simulink model "rule_DJ"  (R2021a)
settings: Solver=FixedStepAuto  StartTime=0.0  StopTime=8.9  FixedStep=1/30  RelTol=1e-3
values from neighbouring files (symbols this model uses):
  y = zeros(10,4)    [simulate.m]
libraries: simulink x17
(part 1 of 3)
settings Model: NumberOfSteps=5  Creator=80720  LastModifiedBy=Administrator
settings SolverCC: AlgebraicLoopSolver=TrustRegion
settings DataIOCC: ReturnWorkspaceOutputs=off
settings DebuggingCC: SFMachineParentedDataDiag=warning  ArithmeticOperatorsInVariantConditions=warning
settings SFSimCC: SimUseLocalCustomCode=off  CustomCodeUndefinedFunction=UseInterfaceOnly
settings RTWCC: RTWUseLocalCustomCode=off

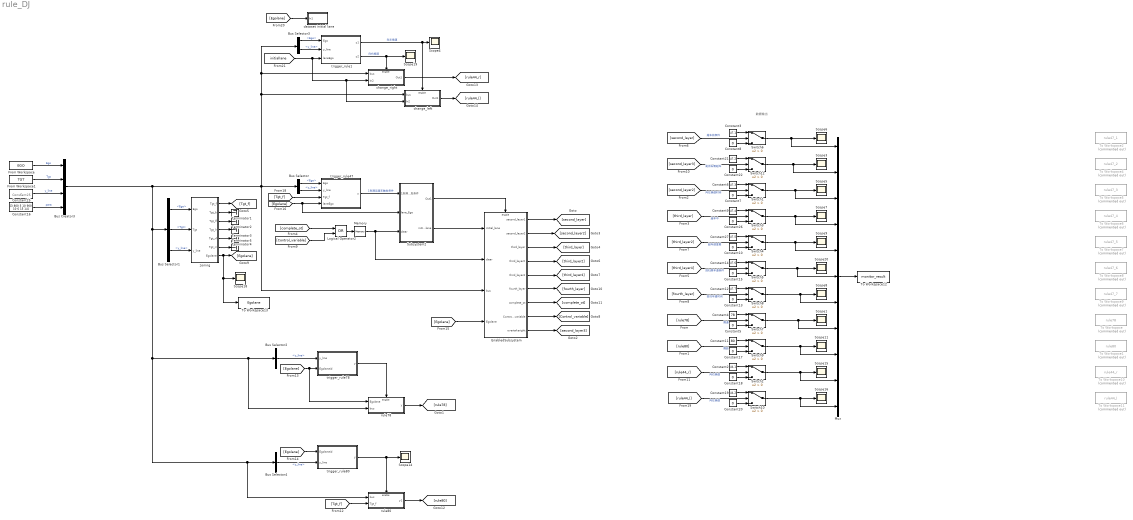
== system rule_DJ ==
  note: Constant25
  note: 数据输出
  Bus Creator3 : BusCreator  Inputs=4
  Bus Selector : BusSelector  OutputSignals=Ego,y_line
  Bus Selector1 : BusSelector  OutputSignals=Ego,Tgt,y_line
  Bus Selector2 : BusSelector  OutputSignals=y_line
  Bus Selector3 : BusSelector  OutputSignals=Ego,y_line
  Bus Selector4 : BusSelector  OutputSignals=y_line
  Constant{5,7..8,10,13,15,17..18,20,22,26} (11 alike) : Constant  Value=0
  Constant11 : Constant  Value=80
  Constant12 : Constant  Value=47.7
  Constant14 : Constant  Value=47.6
  Constant16 : Constant  Value=[3 800 5 10 900 10 6 15 14]
  Constant19 : Constant  Value=44.2
  Constant2 : Constant  Value=44.1
  Constant21 : Constant  Value=47.2
  Constant25 : Constant  Value=y
  Constant27 : Constant  Value=47.5
  Constant3 : Constant  Value=47.1
  Constant4 : Constant  Value=78
  Constant6 : Constant  Value=47.3
  Constant9 : Constant  Value=47.4
  EnabledSubsystem : Subsystem  TreatAsAtomicUnit=on
  From Workspace : FromWorkspace  VariableName=EGO  OutDataTypeStr=Bus: EgoBUS
  From Workspace1 : FromWorkspace  VariableName=TGT  OutDataTypeStr=Bus: TgtBUS
  Logical Operator2 : Logic  Operator=OR  AllPortsSameDT=off  OutDataTypeStr=boolean
  Memory : Memory
  Mux : Mux  Inputs=11
  Scope{1,3..9,11,14..16,18..20} (15 alike) : Scope
  Subsystem2 : Subsystem
  Switch{1..10,12} (11 alike) : Switch  Criteria=u2 > Threshold
  Terminator{1..5} (5 alike) : Terminator
  To Workspace : ToWorkspace  Commented=on  VariableName=rule78  SaveFormat=Timeseries  SampleTime=-1
  To Workspace1 : ToWorkspace  Commented=on  VariableName=rule80  SaveFormat=Timeseries  SampleTime=-1
  To Workspace10 : ToWorkspace  Commented=on  VariableName=rule44_r  SaveFormat=Timeseries  SampleTime=-1
  To Workspace11 : ToWorkspace  Commented=on  VariableName=rule44_l  SaveFormat=Timeseries  SampleTime=-1
  To Workspace12 : ToWorkspace  VariableName=monitor_result  SaveFormat=Timeseries  SampleTime=-1
  To Workspace13 : ToWorkspace  VariableName=Egolane  SaveFormat=Timeseries  SampleTime=-1
  To Workspace2 : ToWorkspace  Commented=on  VariableName=rule47_1  SaveFormat=Timeseries  SampleTime=-1
  To Workspace4 : ToWorkspace  Commented=on  VariableName=rule47_2  SaveFormat=Timeseries  SampleTime=-1
  To Workspace5 : ToWorkspace  Commented=on  VariableName=rule47_3  SaveFormat=Timeseries  SampleTime=-1
  To Workspace6 : ToWorkspace  Commented=on  VariableName=rule47_4  SaveFormat=Timeseries  SampleTime=-1
  To Workspace7 : ToWorkspace  Commented=on  VariableName=rule47_5  SaveFormat=Timeseries  SampleTime=-1
  To Workspace8 : ToWorkspace  Commented=on  VariableName=rule47_6  SaveFormat=Timeseries  SampleTime=-1
  To Workspace9 : ToWorkspace  Commented=on  VariableName=rule47_7  SaveFormat=Timeseries  SampleTime=-1
  change_left : Subsystem  TreatAsAtomicUnit=on
  change_right : Subsystem  TreatAsAtomicUnit=on
  dataset initial lane : Subsystem
  rule78 : Subsystem  TreatAsAtomicUnit=on
  rule80 : Subsystem  TreatAsAtomicUnit=on
  trigger_rule1 : MATLAB Function  TreatAsAtomicUnit=on
  trigger_rule47 : MATLAB Function  TreatAsAtomicUnit=on
  trigger_rule78 : MATLAB Function  TreatAsAtomicUnit=on
  trigger_rule80 : MATLAB Function  TreatAsAtomicUnit=on
  zoning : MATLAB Function  TreatAsAtomicUnit=on
  wires:
  Bus Selector/2 -> trigger_rule47/2(y_line)  "<y_line>"
  Bus Selector/1 -> trigger_rule47/1(Ego)  "<Ego>"
  trigger_rule47/1(y) -> Subsystem2/1(1则满足超车触发条件)  "1则满足超车触发条件"
  Subsystem2/1(Out1) -> EnabledSubsystem/Enable
  Subsystem2/2(initial_lane) -> EnabledSubsystem/1(initial_lane)
  EnabledSubsystem/1(second_layer1) -> [second_layer]
  EnabledSubsystem/3(third_layer) -> [third_layer]
  EnabledSubsystem/4(third_layer2) -> [third_layer2]
  EnabledSubsystem/5(third_layer4) -> [third_layer4]
  EnabledSubsystem/6(fourth_layer) -> [fourth_layer]
  EnabledSubsystem/7(complete_ot) -> [complete_ot]
  EnabledSubsystem/8(Control_variable) -> [Control_variable]
  Constant22/1 -> Switch12/3
  Constant3/1 -> Switch6/1
  Constant13/1 -> Switch8/3
  [fourth_layer] -> Switch8/2  "回归车道时间"
  Constant15/1 -> Switch5/3
  Constant9/1 -> Switch3/1
  Constant21/1 -> Switch12/1
  Switch12/1 -> Mux/2, Scope3/1
  [second_layer3] -> Switch12/2  "是否右侧超车"
  [third_layer2] -> Switch4/2  "超车速度差"
  Constant27/1 -> Switch4/1
  Constant12/1 -> Switch8/1
  Constant10/1 -> Switch4/3
  [third_layer] -> Switch3/2  "超车中"
  [second_layer2] -> Switch1/2  "向左换道时间"
  Constant26/1 -> Switch3/3
  Constant6/1 -> Switch1/1
  Constant7/1 -> Switch1/3
  [second_layer] -> Switch6/2  "超车前条件"
  Constant14/1 -> Switch5/1
  [third_layer4] -> Switch5/2  "回归原车道条件"
  Constant8/1 -> Switch6/3
  Switch6/1 -> Mux/1, Scope6/1
  EnabledSubsystem/9(overtakeright) -> [second_layer3]
  EnabledSubsystem/2(second_layer2) -> [second_layer2]
  From Workspace1/1 -> Bus Creator3/2  "Tgt"
  Constant25/1 -> Bus Creator3/3  "y_line"
  Constant16/1 -> Bus Creator3/4  "para"
  rule78/1(y) -> [rule78]
  trigger_rule78/1(y) -> rule78/Enable
  Bus Selector2/1 -> trigger_rule78/1(y_line)  "<y_line>"
  Bus Selector1/1 -> zoning/1(Ego)  "<Ego>"
  Bus Selector1/2 -> zoning/2(Tgt)  "<Tgt>"
  Bus Selector1/3 -> zoning/3(y_line)  "<y_line>"
  zoning/1(Tgt_f) -> [Tgt_f]
  zoning/2(Tgt_b) -> Terminator1/1
  zoning/3(Tgt_lf) -> Terminator2/1
  zoning/4(Tgt_lr) -> Terminator3/1
  zoning/5(Tgt_rf) -> Terminator4/1
  zoning/6(Tgt_rr) -> Terminator5/1
  [Tgt_f] -> trigger_rule47/3(Tgt_f)
  [Control_variable] -> Logical Operator2/2
  [complete_ot] -> Logical Operator2/1
  Logical Operator2/1 -> Memory/1
  Memory/1 -> EnabledSubsystem/2(clear), Subsystem2/3(clear)
  Bus Selector4/1 -> trigger_rule80/2(y_line)  "<y_line>"
  trigger_rule80/1(y) -> rule80/Enable, Scope14/1
  [Tgt_f] -> rule80/2(Tgt_f)
  zoning/7(Egolane) -> To Workspace13/1, Scope18/1, [Egolane]
  [Egolane] -> rule78/1(Egolane), trigger_rule78/2(Egolaneid)
  [Egolane] -> trigger_rule80/1(Egolaneid)
  [Egolane] -> Subsystem2/2(lane_Ego), trigger_rule47/4(laneEgo)
  [Egolane] -> EnabledSubsystem/4(Egolane)
  From Workspace/1 -> Bus Creator3/1  "Ego"
  Bus Creator3/1 -> Bus Selector1/1, rule80/1(bus), Bus Selector4/1, rule78/2(bus), Bus Selector2/1, change_right/1(bus), Bus Selector3/1, change_left/1(bus), Bus Selector/1, EnabledSubsystem/3(bus)
  Bus Selector3/1 -> trigger_rule1/1(Ego)  "<Ego>"
  Bus Selector3/2 -> trigger_rule1/2(y_line)  "<y_line>"
  [initiallane] -> change_left/2(In2), change_right/2(In2), trigger_rule1/3(laneEgo)
  trigger_rule1/1(y1) -> change_left/Enable, Scope4/1  "向左换道"
  trigger_rule1/2(y2) -> change_right/Enable, Scope19/1  "向右换道"
  Switch3/1 -> Mux/4, Scope7/1
  Switch4/1 -> Mux/5, Scope9/1
  Switch5/1 -> Mux/6, Scope20/1
  Switch8/1 -> Mux/7, Scope8/1
  Switch1/1 -> Mux/3, Scope5/1
  Constant5/1 -> Switch7/3
  Constant4/1 -> Switch7/1
  [rule78] -> Switch7/2  "限速"
  rule80/1(y1) -> [rule80]
  Constant11/1 -> Switch9/1
  [rule80] -> Switch9/2  "限距"
  Constant17/1 -> Switch9/3
  Switch7/1 -> Mux/8, Scope1/1
  Switch9/1 -> Mux/9, Scope11/1
  change_right/1(Out1) -> [rule44_r]
  change_left/1(Out1) -> [rule44_l]
  Switch2/1 -> Mux/10, Scope15/1
  Constant2/1 -> Switch2/1
  Constant18/1 -> Switch2/3
  [rule44_r] -> Switch2/2  "向右换道"
  Switch10/1 -> Mux/11, Scope16/1
  Constant19/1 -> Switch10/1
  Constant20/1 -> Switch10/3
  [rule44_l] -> Switch10/2  "向左换道"
  Mux/1 -> To Workspace12/1
  [Egolane] -> dataset initial lane/1(In1)

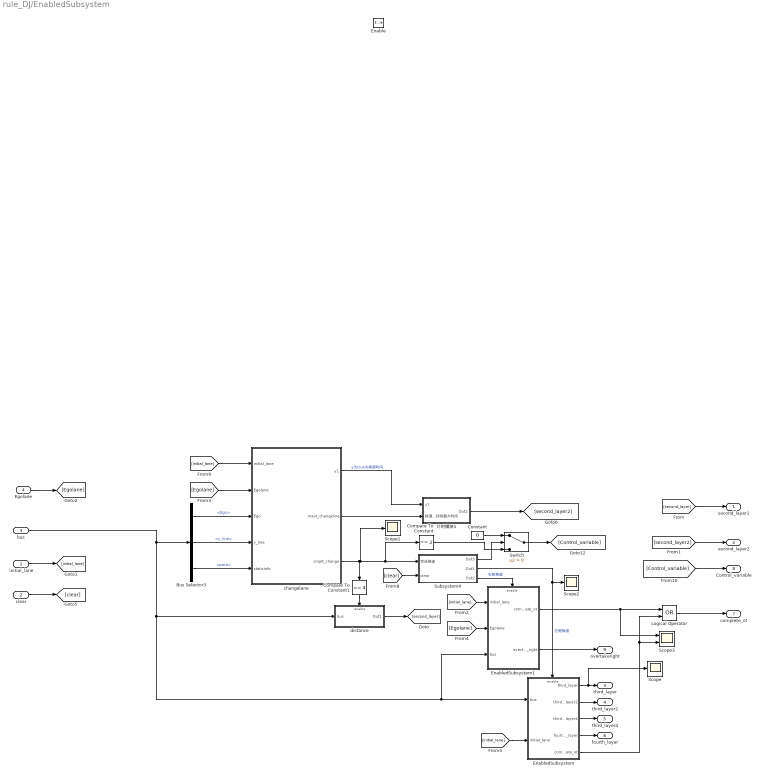
== system rule_DJ/EnabledSubsystem ==
  initial_lane : Inport
  clear : Inport  Port=2
  bus : Inport  Port=3
  Egolane : Inport  Port=4
  Enable : EnablePort
  Bus Selector3 : BusSelector  OutputSignals=Ego,y_line,para
  Compare To Constant : simulink/Logic and Bit Operations/Compare To Constant  relop===  const=2  OutDataTypeStr=boolean
  Compare To Constant1 : simulink/Logic and Bit Operations/Compare To Constant  relop===  const=4  OutDataTypeStr=boolean
  Constant : Constant  Value=0
  EnabledSubsystem : Subsystem  TreatAsAtomicUnit=on
  EnabledSubsystem1 : Subsystem  TreatAsAtomicUnit=on
  Logical Operator : Logic  Operator=OR  AllPortsSameDT=off  OutDataTypeStr=boolean
  Scope : Scope
  Scope1 : Scope
  Scope2 : Scope
  Scope3 : Scope  NumInputPorts=2
  Subsystem4 : Subsystem
  Switch : Switch  Criteria=u2 > Threshold
  changelane : MATLAB Function  TreatAsAtomicUnit=on
  distance : Subsystem  TreatAsAtomicUnit=on
  计时模块1 : Subsystem
  second_layer1 : Outport  OutputWhenDisabled=reset  InitialOutput=0
  second_layer2 : Outport  Port=2  OutputWhenDisabled=reset  InitialOutput=0
  third_layer : Outport  Port=3  OutputWhenDisabled=reset  InitialOutput=0
  third_layer2 : Outport  Port=4  OutputWhenDisabled=reset  InitialOutput=0
  third_layer4 : Outport  Port=5  OutputWhenDisabled=reset  InitialOutput=0
  fourth_layer : Outport  Port=6  OutputWhenDisabled=reset  InitialOutput=0
  complete_ot : Outport  Port=7  OutputWhenDisabled=reset  InitialOutput=0
  Control_variable : Outport  Port=8  OutputWhenDisabled=reset  InitialOutput=0
  overtakeright : Outport  Port=9  OutputWhenDisabled=reset  InitialOutput=0
  wires:
  EnabledSubsystem/1(third_layer) -> Scope/1, third_layer/1
  EnabledSubsystem/4(fourth_layer) -> fourth_layer/1
  EnabledSubsystem/3(third_layer4) -> third_layer4/1
  EnabledSubsystem/2(third_layer2) -> third_layer2/1
  initial_lane/1 -> [initial_lane]
  clear/1 -> [clear]
  [initial_lane] -> EnabledSubsystem/2(initial_lane)
  [second_layer] -> second_layer1/1
  [second_layer2] -> second_layer2/1
  bus/1 -> EnabledSubsystem1/3(bus), EnabledSubsystem/1(bus), distance/1(bus), Bus Selector3/1
  changelane/1(y1) -> 计时模块1/1(y1)  "y为true为换道时间"
  [clear] -> Subsystem4/2(clear)
  Bus Selector3/2 -> changelane/4(y_line)  "<y_line>"
  [initial_lane] -> changelane/1(initial_lane)
  changelane/2(maxt_changeline) -> 计时模块1/2(换道持续最大时间)
  Subsystem4/2(Out1) -> Scope2/1, EnabledSubsystem/Enable  "左侧换道"
  Bus Selector3/1 -> changelane/3(Ego)  "<Ego>"
  distance/1(Out1) -> [second_layer]
  [Control_variable] -> Control_variable/1
  计时模块1/1(Out2) -> [second_layer2]
  Bus Selector3/3 -> changelane/5(staticinfo)  "<para>"
  Compare To Constant1/1 -> distance/Enable
  changelane/3(cmplt_change) -> Scope1/1, Compare To Constant/1, Subsystem4/1(完成换道), Compare To Constant1/1
  Subsystem4/3(Out2) -> EnabledSubsystem1/Enable  "右侧换道"
  [initial_lane] -> EnabledSubsystem1/1(initial_lane)
  Egolane/1 -> [Egolane]
  [Egolane] -> changelane/2(Egolane)
  [Egolane] -> EnabledSubsystem1/2(Egolane)
  EnabledSubsystem1/1(complete_ot) -> Scope3/1, Logical Operator/1
  EnabledSubsystem/5(complete_ot) -> Scope3/2, Logical Operator/2
  Logical Operator/1 -> complete_ot/1
  EnabledSubsystem1/2(overtake_right) -> overtakeright/1
  Subsystem4/1(Out3) -> Switch/2
  Compare To Constant/1 -> Switch/3
  Switch/1 -> [Control_variable]
  Constant/1 -> Switch/1

== system rule_DJ/Subsystem2 ==
  1则满足超车触发条件 : Inport
  lane_Ego : Inport  Port=2
  clear : Inport  Port=3
  Triggered Subsystem2 : Subsystem  TreatAsAtomicUnit=on
  使能信号生成 : Subsystem
  Out1 : Outport  VectorParamsAs1DForOutWhenUnconnected=off
  initial_lane : Outport  Port=2  VectorParamsAs1DForOutWhenUnconnected=off
  wires:
  使能信号生成/1(enable) -> Triggered Subsystem2/Trigger, Out1/1  "输出为1，满足超车监测条件"
  Triggered Subsystem2/1(Out1) -> initial_lane/1
  clear/1 -> 使能信号生成/2(cons)
  lane_Ego/1 -> Triggered Subsystem2/1(lane_Ego)
  1则满足超车触发条件/1 -> 使能信号生成/1(pros)

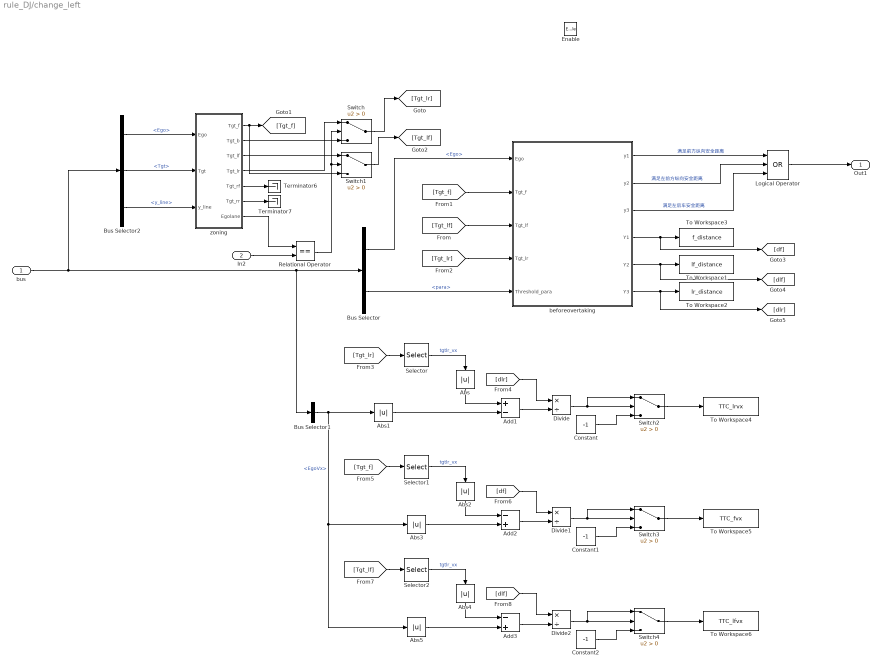
== system rule_DJ/change_left ==
  bus : Inport
  In2 : Inport  Port=2
  Enable : EnablePort  StatesWhenEnabling=reset
  Abs{,1..5} (6 alike) : Abs
  Add1 : Sum  Inputs=+-
  Add2 : Sum  Inputs=-+
  Add3 : Sum  Inputs=-+
  Bus Selector : BusSelector  OutputSignals=Ego,para
  Bus Selector1 : BusSelector  OutputSignals=Ego.EgoVx
  Bus Selector2 : BusSelector  OutputSignals=Ego,Tgt,y_line
  Constant : Constant  Value=-1
  Constant1 : Constant  Value=-1
  Constant2 : Constant  Value=-1
  Divide : Product  Inputs=*/
  Divide1 : Product  Inputs=*/
  Divide2 : Product  Inputs=*/
  Logical Operator : Logic  Operator=OR  Inputs=3  AllPortsSameDT=off  OutDataTypeStr=boolean
  Relational Operator : RelationalOperator  Operator===  OutDataTypeStr=boolean  RndMeth=Simplest
  Selector : Selector  InputPortWidth=5  IndexOptions=Index vector (dialog)  Indices=[3]  OutputSizes=1
  Selector1 : Selector  InputPortWidth=5  IndexOptions=Index vector (dialog)  Indices=[3]  OutputSizes=1
  Selector2 : Selector  InputPortWidth=5  IndexOptions=Index vector (dialog)  Indices=[3]  OutputSizes=1
  Switch{,1..4} (5 alike) : Switch  Criteria=u2 > Threshold
  Terminator6 : Terminator
  Terminator7 : Terminator
  To Workspace1 : ToWorkspace  VariableName=lf_distance  SaveFormat=Timeseries  SampleTime=-1
  To Workspace2 : ToWorkspace  VariableName=lr_distance  SaveFormat=Timeseries  SampleTime=-1
  To Workspace3 : ToWorkspace  VariableName=f_distance  SaveFormat=Timeseries  SampleTime=-1
  To Workspace4 : ToWorkspace  VariableName=TTC_lrvx  SaveFormat=Timeseries  SampleTime=-1
  To Workspace5 : ToWorkspace  VariableName=TTC_fvx  SaveFormat=Timeseries  SampleTime=-1
  To Workspace6 : ToWorkspace  VariableName=TTC_lfvx  SaveFormat=Timeseries  SampleTime=-1
  beforeovertaking : MATLAB Function  TreatAsAtomicUnit=on
  zoning : MATLAB Function  TreatAsAtomicUnit=on
  Out1 : Outport  OutputWhenDisabled=reset  InitialOutput=0
  wires:
  beforeovertaking/3(y3) -> Logical Operator/3  "满足左后车安全距离"
  beforeovertaking/1(y1) -> Logical Operator/1  "满足前方纵向安全距离"
  [Tgt_lf] -> beforeovertaking/3(Tgt_lf)
  beforeovertaking/2(y2) -> Logical Operator/2  "满足左前方纵向安全距离"
  [Tgt_lr] -> beforeovertaking/4(Tgt_lr)
  bus/1 -> Bus Selector2/1, Bus Selector/1, Bus Selector1/1
  Bus Selector2/1 -> zoning/1(Ego)  "<Ego>"
  Bus Selector2/2 -> zoning/2(Tgt)  "<Tgt>"
  Bus Selector2/3 -> zoning/3(y_line)  "<y_line>"
  [Tgt_f] -> beforeovertaking/2(Tgt_f)
  Bus Selector/1 -> beforeovertaking/1(Ego)  "<Ego>"
  Bus Selector/2 -> beforeovertaking/5(Threshold_para)  "<para>"
  beforeovertaking/4(Y1) -> [df], To Workspace3/1
  beforeovertaking/5(Y2) -> [dlf], To Workspace1/1
  beforeovertaking/6(Y3) -> [dlr], To Workspace2/1
  zoning/5(Tgt_rf) -> Terminator6/1
  zoning/7(Egolane) -> Relational Operator/1
  zoning/2(Tgt_b) -> Switch/3
  zoning/1(Tgt_f) -> Switch1/3, [Tgt_f]
  zoning/6(Tgt_rr) -> Terminator7/1
  zoning/3(Tgt_lf) -> Switch1/1
  zoning/4(Tgt_lr) -> Switch/1
  Logical Operator/1 -> Out1/1
  In2/1 -> Relational Operator/2
  Relational Operator/1 -> Switch/2, Switch1/2
  Switch/1 -> [Tgt_lr]
  Switch1/1 -> [Tgt_lf]
  Constant1/1 -> Switch3/3
  Bus Selector1/1 -> Abs5/1, Abs3/1, Abs1/1  "<EgoVx>"
  Abs1/1 -> Add1/2
  Abs/1 -> Add1/1
  Add3/1 -> Divide2/2
  Constant/1 -> Switch2/3
  Switch4/1 -> To Workspace6/1
  [dlf] -> Divide2/1
  Abs4/1 -> Add3/1
  [Tgt_lr] -> Selector/1
  Switch2/1 -> To Workspace4/1
  Constant2/1 -> Switch4/3
  Selector/1 -> Abs/1  "tgtlr_vx"
  Add1/1 -> Divide/2
  Abs2/1 -> Add2/1
  [Tgt_lf] -> Selector2/1
  Add2/1 -> Divide1/2
  Abs3/1 -> Add2/2
  Divide1/1 -> Switch3/1, Switch3/2
  Switch3/1 -> To Workspace5/1
  Abs5/1 -> Add3/2
  [Tgt_f] -> Selector1/1
  Divide/1 -> Switch2/1, Switch2/2
  Selector1/1 -> Abs2/1  "tgtlr_vx"
  [df] -> Divide1/1
  Selector2/1 -> Abs4/1  "tgtlr_vx"
  [dlr] -> Divide/1
  Divide2/1 -> Switch4/1, Switch4/2

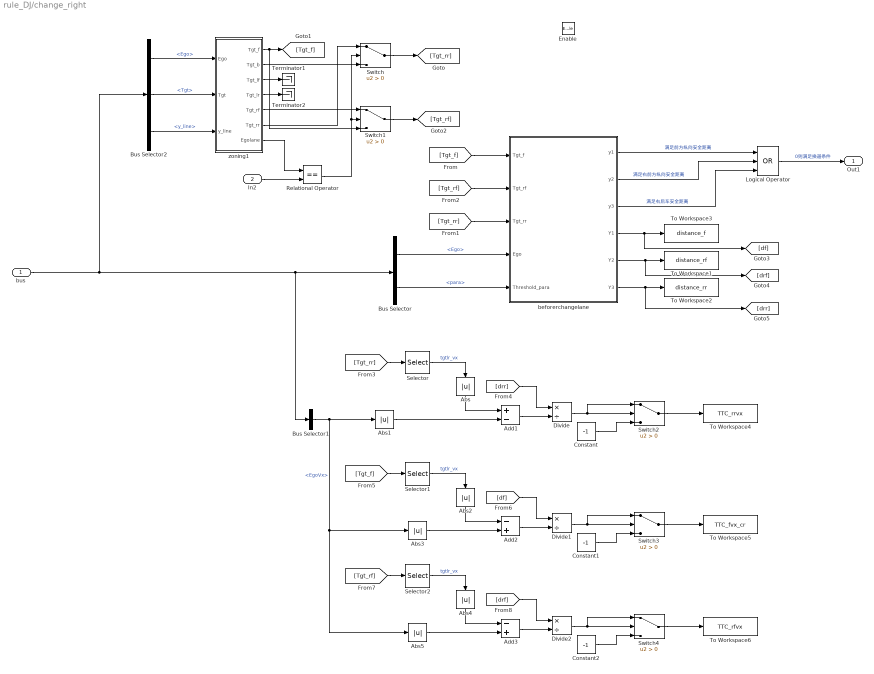
== system rule_DJ/change_right ==
  bus : Inport
  In2 : Inport  Port=2
  Enable : EnablePort  StatesWhenEnabling=reset
  Abs{,1..5} (6 alike) : Abs
  Add1 : Sum  Inputs=+-
  Add2 : Sum  Inputs=-+
  Add3 : Sum  Inputs=-+
  Bus Selector : BusSelector  OutputSignals=Ego,para
  Bus Selector1 : BusSelector  OutputSignals=Ego.EgoVx
  Bus Selector2 : BusSelector  OutputSignals=Ego,Tgt,y_line
  Constant : Constant  Value=-1
  Constant1 : Constant  Value=-1
  Constant2 : Constant  Value=-1
  Divide : Product  Inputs=*/
  Divide1 : Product  Inputs=*/
  Divide2 : Product  Inputs=*/
  Logical Operator : Logic  Operator=OR  Inputs=3  AllPortsSameDT=off  OutDataTypeStr=boolean
  Relational Operator : RelationalOperator  Operator===  OutDataTypeStr=boolean  RndMeth=Simplest
  Selector : Selector  InputPortWidth=5  IndexOptions=Index vector (dialog)  Indices=[3]  OutputSizes=1
  Selector1 : Selector  InputPortWidth=5  IndexOptions=Index vector (dialog)  Indices=[3]  OutputSizes=1
  Selector2 : Selector  InputPortWidth=5  IndexOptions=Index vector (dialog)  Indices=[3]  OutputSizes=1
  Switch{,1..4} (5 alike) : Switch  Criteria=u2 > Threshold
  Terminator1 : Terminator
  Terminator2 : Terminator
  To Workspace1 : ToWorkspace  VariableName=distance_rf  SaveFormat=Timeseries  SampleTime=-1
  To Workspace2 : ToWorkspace  VariableName=distance_rr  SaveFormat=Timeseries  SampleTime=-1
  To Workspace3 : ToWorkspace  VariableName=distance_f  SaveFormat=Timeseries  SampleTime=-1
  To Workspace4 : ToWorkspace  VariableName=TTC_rrvx  SaveFormat=Timeseries  SampleTime=-1
  To Workspace5 : ToWorkspace  VariableName=TTC_fvx_cr  SaveFormat=Timeseries  SampleTime=-1
  To Workspace6 : ToWorkspace  VariableName=TTC_rfvx  SaveFormat=Timeseries  SampleTime=-1
  beforerchangelane : MATLAB Function  TreatAsAtomicUnit=on
  zoning1 : MATLAB Function  TreatAsAtomicUnit=on
  Out1 : Outport  OutputWhenDisabled=reset  InitialOutput=0
  wires:
  beforerchangelane/3(y3) -> Logical Operator/3  "满足右后车安全距离"
  Logical Operator/1 -> Out1/1  "0则满足换道条件"
  beforerchangelane/1(y1) -> Logical Operator/1  "满足前方纵向安全距离"
  beforerchangelane/2(y2) -> Logical Operator/2  "满足右前方纵向安全距离"
  Bus Selector2/1 -> zoning1/1(Ego)  "<Ego>"
  Bus Selector2/2 -> zoning1/2(Tgt)  "<Tgt>"
  Bus Selector2/3 -> zoning1/3(y_line)  "<y_line>"
  Bus Selector/1 -> beforerchangelane/4(Ego)  "<Ego>"
  Bus Selector/2 -> beforerchangelane/5(Threshold_para)  "<para>"
  Relational Operator/1 -> Switch/2, Switch1/2
  Switch/1 -> [Tgt_rr]
  zoning1/2(Tgt_b) -> Switch/3
  Switch1/1 -> [Tgt_rf]
  zoning1/6(Tgt_rr) -> Switch/1
  zoning1/1(Tgt_f) -> Switch1/3, [Tgt_f]
  zoning1/7(Egolane) -> Relational Operator/1
  zoning1/5(Tgt_rf) -> Switch1/1
  In2/1 -> Relational Operator/2
  zoning1/3(Tgt_lf) -> Terminator1/1
  zoning1/4(Tgt_lr) -> Terminator2/1
  [Tgt_f] -> beforerchangelane/1(Tgt_f)
  [Tgt_rf] -> beforerchangelane/2(Tgt_rf)
  [Tgt_rr] -> beforerchangelane/3(Tgt_rr)
  bus/1 -> Bus Selector1/1, Bus Selector/1, Bus Selector2/1
  beforerchangelane/4(Y1) -> [df], To Workspace3/1
  beforerchangelane/6(Y3) -> [drr], To Workspace2/1
  beforerchangelane/5(Y2) -> [drf], To Workspace1/1
  Abs/1 -> Add1/1
  Divide/1 -> Switch2/1, Switch2/2
  [drr] -> Divide/1
  Divide2/1 -> Switch4/1, Switch4/2
  Abs3/1 -> Add2/2
  Selector1/1 -> Abs2/1  "tgtlr_vx"
  [Tgt_f] -> Selector1/1
  [Tgt_rr] -> Selector/1
  Abs1/1 -> Add1/2
  Abs5/1 -> Add3/2
  Bus Selector1/1 -> Abs5/1, Abs3/1, Abs1/1  "<EgoVx>"
  Selector2/1 -> Abs4/1  "tgtlr_vx"
  Abs4/1 -> Add3/1
  Switch4/1 -> To Workspace6/1
  Add1/1 -> Divide/2
  Constant/1 -> Switch2/3
  Constant1/1 -> Switch3/3
  Divide1/1 -> Switch3/1, Switch3/2
  [df] -> Divide1/1
  Add3/1 -> Divide2/2
  Abs2/1 -> Add2/1
  Selector/1 -> Abs/1  "tgtlr_vx"
  Switch2/1 -> To Workspace4/1
  [drf] -> Divide2/1
  Add2/1 -> Divide1/2
  Constant2/1 -> Switch4/3
  Switch3/1 -> To Workspace5/1
  [Tgt_rf] -> Selector2/1

== system rule_DJ/dataset initial lane ==
  In1 : Inport
  Clock : Clock
  Compare To Zero : simulink/Logic and Bit Operations/Compare To Zero  relop=>  OutDataTypeStr=boolean
  Scope13 : Scope
  Switch : Switch  Criteria=u2 > Threshold
  Triggered Subsystem : Subsystem  TreatAsAtomicUnit=on
  tag scope: initiallane=global
  wires:
  Clock/1 -> Compare To Zero/1
  Compare To Zero/1 -> Triggered Subsystem/Trigger, Scope13/1
  Switch/1 -> [initiallane]
  In1/1 -> Switch/3, Triggered Subsystem/1(In1)
  Triggered Subsystem/1(Out1) -> Switch/2, Switch/1

== system rule_DJ/rule78 ==
  Egolane : Inport
  bus : Inport  Port=2
  Enable : EnablePort  StatesWhenEnabling=reset
  Bus Selector : BusSelector  OutputSignals=Ego.EgoX,para
  Bus Selector2 : BusSelector  OutputSignals=Ego.EgoX,Ego.EgoVx,para
  Compliance Speed : ToWorkspace  VariableName=Cs  SaveFormat=Timeseries  SampleTime=-1
  进入限速标志管理区域判断 : MATLAB Function  TreatAsAtomicUnit=on
  限速标志管理区域 : Subsystem
  高速限速监测 : MATLAB Function  TreatAsAtomicUnit=on
  y : Outport  OutputWhenDisabled=reset  InitialOutput=0
  wires:
  进入限速标志管理区域判断/1(Enter_spdlimit_section) -> 限速标志管理区域/1(Enter)
  限速标志管理区域/1(spdsign_section) -> 高速限速监测/5(spdsign_section)  "1为处于限速标志区域"
  Bus Selector/2 -> 进入限速标志管理区域判断/2(staticinfo)  "<para>"
  高速限速监测/2(clear) -> 限速标志管理区域/2(clear)
  bus/1 -> Bus Selector2/1, Bus Selector/1
  Bus Selector/1 -> 进入限速标志管理区域判断/1(Egox)  "<EgoX>"
  Bus Selector2/1 -> 高速限速监测/2(Egox)  "<EgoX>"
  Bus Selector2/2 -> 高速限速监测/3(Egovx)  "<EgoVx>"
  Bus Selector2/3 -> 高速限速监测/4(staticinfo)  "<para>"
  Egolane/1 -> 高速限速监测/1(Egolaneid)
  高速限速监测/1(y) -> y/1
  高速限速监测/3(Cs) -> Compliance Speed/1

== system rule_DJ/rule80 ==
  bus : Inport
  Tgt_f : Inport  Port=2
  Enable : EnablePort  StatesWhenEnabling=reset
  Bus Selector : BusSelector  OutputSignals=Ego
  To Workspace1 : ToWorkspace  VariableName=Cd  SaveFormat=Timeseries  SampleTime=-1
  To Workspace3 : ToWorkspace  VariableName=distance  SaveFormat=Timeseries  SampleTime=-1
  高速保持车距监测 : MATLAB Function  TreatAsAtomicUnit=on
  y1 : Outport  OutputWhenDisabled=reset  InitialOutput=0
  wires:
  bus/1 -> Bus Selector/1
  Bus Selector/1 -> 高速保持车距监测/1(Ego)  "<Ego>"
  Tgt_f/1 -> 高速保持车距监测/2(Tgt_f)
  高速保持车距监测/1(y) -> y1/1
  高速保持车距监测/2(y2) -> To Workspace3/1
  高速保持车距监测/3(Cd) -> To Workspace1/1

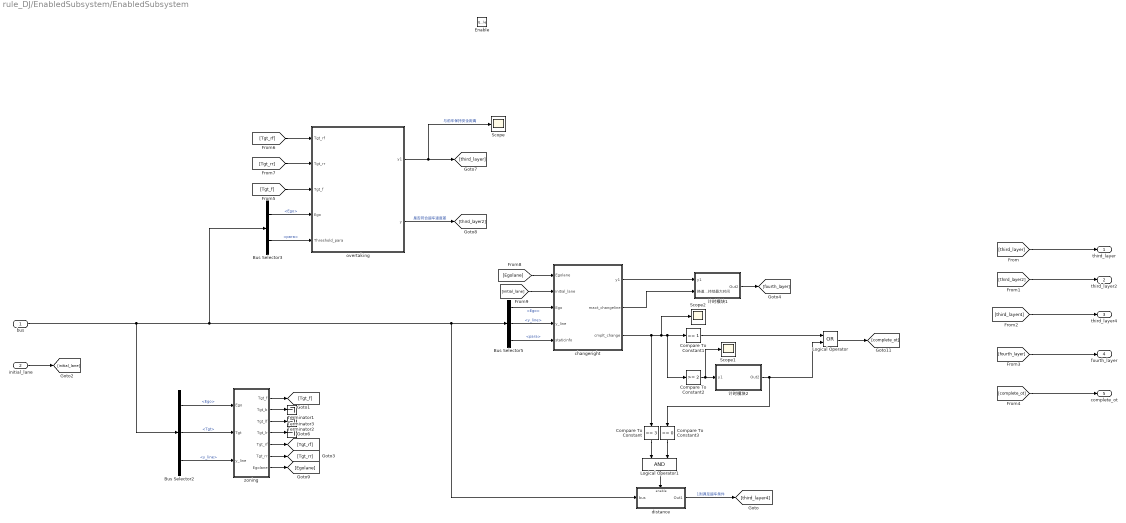
== system rule_DJ/EnabledSubsystem/EnabledSubsystem ==
  bus : Inport
  initial_lane : Inport  Port=2
  Enable : EnablePort
  Bus Selector2 : BusSelector  OutputSignals=Ego,Tgt,y_line
  Bus Selector3 : BusSelector  OutputSignals=Ego,para
  Bus Selector5 : BusSelector  OutputSignals=Ego,y_line,para
  Compare To Constant : simulink/Logic and Bit Operations/Compare To Constant  relop===  const=3  OutDataTypeStr=boolean
  Compare To Constant1 : simulink/Logic and Bit Operations/Compare To Constant  relop===  const=1  OutDataTypeStr=boolean
  Compare To Constant2 : simulink/Logic and Bit Operations/Compare To Constant  relop=>=  const=2  OutDataTypeStr=boolean
  Compare To Constant3 : simulink/Logic and Bit Operations/Compare To Constant  relop===  const=0  OutDataTypeStr=boolean
  Logical Operator : Logic  Operator=OR  AllPortsSameDT=off  OutDataTypeStr=boolean
  Logical Operator1 : Logic  AllPortsSameDT=off  OutDataTypeStr=boolean
  Scope : Scope
  Scope1 : Scope
  Scope2 : Scope
  Terminator1 : Terminator
  Terminator2 : Terminator
  Terminator3 : Terminator
  changeright : MATLAB Function  TreatAsAtomicUnit=on
  distance : Subsystem  TreatAsAtomicUnit=on
  overtaking : MATLAB Function  TreatAsAtomicUnit=on
  zoning : MATLAB Function  TreatAsAtomicUnit=on
  计时模块1 : Subsystem
  计时模块2 : Subsystem
  third_layer : Outport  OutputWhenDisabled=reset  InitialOutput=0
  third_layer2 : Outport  Port=2  OutputWhenDisabled=reset  InitialOutput=0
  third_layer4 : Outport  Port=3  OutputWhenDisabled=reset  InitialOutput=0
  fourth_layer : Outport  Port=4  OutputWhenDisabled=reset  InitialOutput=0
  complete_ot : Outport  Port=5  OutputWhenDisabled=reset  InitialOutput=0
  wires:
  overtaking/2(y) -> [third_layer2]  "是否符合超车速度差"
  Bus Selector3/1 -> overtaking/4(Ego)  "<Ego>"
  Bus Selector5/1 -> changeright/3(Ego)  "<Ego>"
  changeright/1(y1) -> 计时模块1/1(y1)
  distance/1(Out1) -> [third_layer4]  "1则满足超车条件"
  Bus Selector3/2 -> overtaking/5(Threshold_para)  "<para>"
  overtaking/1(y1) -> Scope/1, [third_layer]  "与前车保持安全距离"
  [initial_lane] -> changeright/2(initial_lane)
  changeright/2(maxt_changeline) -> 计时模块1/2(换道持续最大时间)
  initial_lane/1 -> [initial_lane]
  [third_layer] -> third_layer/1
  [third_layer2] -> third_layer2/1
  [third_layer4] -> third_layer4/1
  [fourth_layer] -> fourth_layer/1
  [complete_ot] -> complete_ot/1
  计时模块1/1(Out2) -> [fourth_layer]
  Bus Selector2/2 -> zoning/2(Tgt)  "<Tgt>"
  bus/1 -> Bus Selector2/1, distance/1(bus), Bus Selector5/1, Bus Selector3/1
  Bus Selector2/3 -> zoning/3(y_line)  "<y_line>"
  Bus Selector2/1 -> zoning/1(Ego)  "<Ego>"
  [Tgt_f] -> overtaking/3(Tgt_f)
  [Tgt_rr] -> overtaking/2(Tgt_rr)
  [Tgt_rf] -> overtaking/1(Tgt_rf)
  Bus Selector5/2 -> changeright/4(y_line)  "<y_line>"
  Bus Selector5/3 -> changeright/5(staticinfo)  "<para>"
  Compare To Constant/1 -> Logical Operator1/1
  Logical Operator1/1 -> distance/Enable
  changeright/3(cmplt_change) -> Compare To Constant/1, Scope2/1, Compare To Constant2/1, Compare To Constant1/1
  zoning/5(Tgt_rf) -> [Tgt_rf]
  zoning/4(Tgt_lr) -> Terminator3/1
  zoning/7(Egolane) -> [Egolane]
  zoning/3(Tgt_lf) -> Terminator2/1
  zoning/2(Tgt_b) -> Terminator1/1
  zoning/1(Tgt_f) -> [Tgt_f]
  zoning/6(Tgt_rr) -> [Tgt_rr]
  [Egolane] -> changeright/1(Egolane)
  Compare To Constant2/1 -> 计时模块2/1(y1), Scope1/1
  Compare To Constant3/1 -> Logical Operator1/2
  Compare To Constant1/1 -> Logical Operator/1
  Logical Operator/1 -> [complete_ot]
  计时模块2/1(Out2) -> Logical Operator/2, Compare To Constant3/1

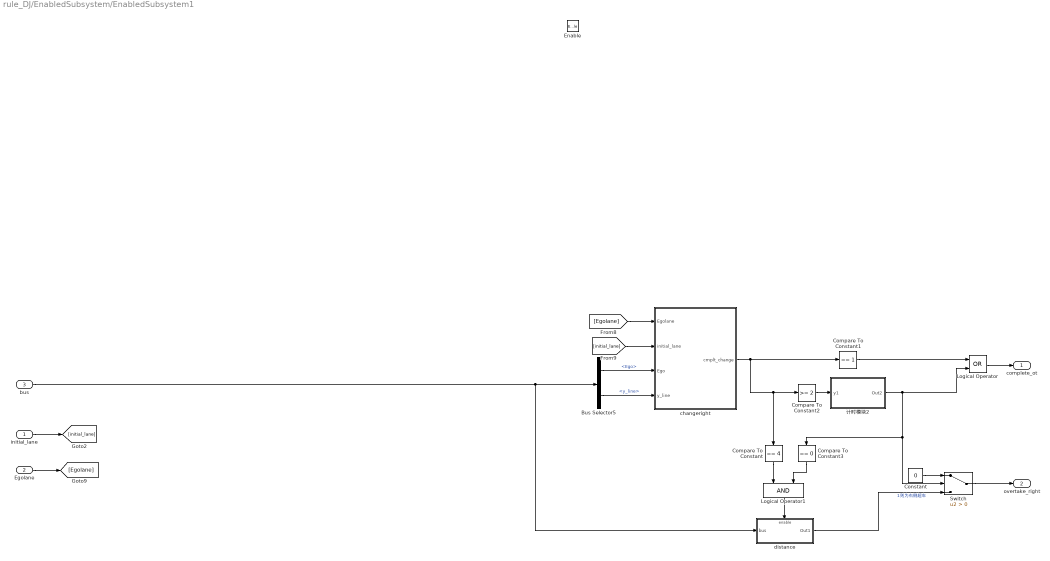
== system rule_DJ/EnabledSubsystem/EnabledSubsystem1 ==
  initial_lane : Inport
  Egolane : Inport  Port=2
  bus : Inport  Port=3
  Enable : EnablePort
  Bus Selector5 : BusSelector  OutputSignals=Ego,y_line
  Compare To Constant : simulink/Logic and Bit Operations/Compare To Constant  relop===  const=4  OutDataTypeStr=boolean
  Compare To Constant1 : simulink/Logic and Bit Operations/Compare To Constant  relop===  const=1  OutDataTypeStr=boolean
  Compare To Constant2 : simulink/Logic and Bit Operations/Compare To Constant  relop=>=  const=2  OutDataTypeStr=boolean
  Compare To Constant3 : simulink/Logic and Bit Operations/Compare To Constant  relop===  const=0  OutDataTypeStr=boolean
  Constant : Constant  Value=0
  Logical Operator : Logic  Operator=OR  AllPortsSameDT=off  OutDataTypeStr=boolean
  Logical Operator1 : Logic  AllPortsSameDT=off  OutDataTypeStr=boolean
  Switch : Switch  Criteria=u2 > Threshold
  changeright : MATLAB Function  TreatAsAtomicUnit=on
  distance : Subsystem  TreatAsAtomicUnit=on
  计时模块2 : Subsystem
  complete_ot : Outport  OutputWhenDisabled=reset  InitialOutput=0
  overtake_right : Outport  Port=2  OutputWhenDisabled=reset  InitialOutput=0
  wires:
  Compare To Constant3/1 -> Logical Operator1/2
  Compare To Constant2/1 -> 计时模块2/1(y1)
  [Egolane] -> changeright/1(Egolane)
  changeright/1(cmplt_change) -> Compare To Constant/1, Compare To Constant2/1, Compare To Constant1/1
  Logical Operator1/1 -> distance/Enable
  Compare To Constant/1 -> Logical Operator1/1
  Bus Selector5/2 -> changeright/4(y_line)  "<y_line>"
  bus/1 -> Bus Selector5/1, distance/1(bus)
  Logical Operator/1 -> complete_ot/1
  initial_lane/1 -> [initial_lane]
  [initial_lane] -> changeright/2(initial_lane)
  Bus Selector5/1 -> changeright/3(Ego)  "<Ego>"
  distance/1(Out1) -> Switch/3  "1则为右侧超车"
  Constant/1 -> Switch/1
  Switch/1 -> overtake_right/1
  Egolane/1 -> [Egolane]
  计时模块2/1(Out2) -> Logical Operator/2, Switch/2, Compare To Constant3/1
  Compare To Constant1/1 -> Logical Operator/1

== system rule_DJ/EnabledSubsystem/Subsystem4 ==
  完成换道 : Inport
  clear : Inport  Port=2
  Compare To Constant : simulink/Logic and Bit Operations/Compare To Constant  relop===  const=1  OutDataTypeStr=boolean
  Compare To Constant1 : simulink/Logic and Bit Operations/Compare To Constant  relop===  const=3  OutDataTypeStr=boolean
  Logical Operator : Logic  Operator=OR  AllPortsSameDT=off  OutDataTypeStr=boolean
  使能信号生成 : Subsystem
  使能信号生成1 : Subsystem
  Out3 : Outport  VectorParamsAs1DForOutWhenUnconnected=off
  Out1 : Outport  Port=2  VectorParamsAs1DForOutWhenUnconnected=off
  Out2 : Outport  Port=3  VectorParamsAs1DForOutWhenUnconnected=off
  wires:
  clear/1 -> 使能信号生成1/2(cons), 使能信号生成/2(cons)
  使能信号生成/1(enable) -> Out1/1, Logical Operator/1
  Compare To Constant/1 -> 使能信号生成/1(pros)
  完成换道/1 -> Compare To Constant1/1, Compare To Constant/1
  使能信号生成1/1(enable) -> Out2/1, Logical Operator/2
  Compare To Constant1/1 -> 使能信号生成1/1(pros)
  Logical Operator/1 -> Out3/1

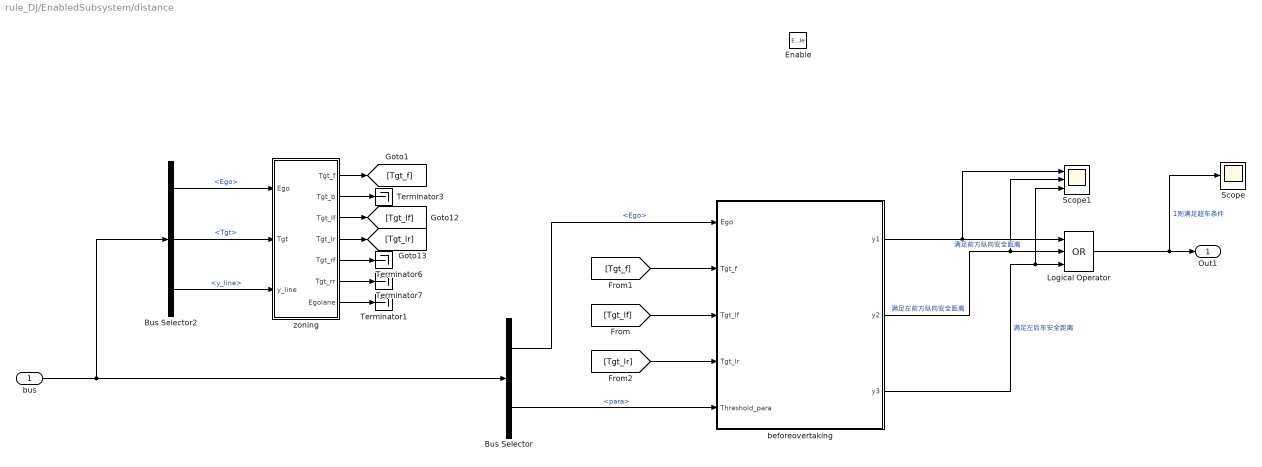
== system rule_DJ/EnabledSubsystem/distance ==
  bus : Inport
  Enable : EnablePort  StatesWhenEnabling=reset
  Bus Selector : BusSelector  OutputSignals=Ego,para
  Bus Selector2 : BusSelector  OutputSignals=Ego,Tgt,y_line
  Logical Operator : Logic  Operator=OR  Inputs=3  AllPortsSameDT=off  OutDataTypeStr=boolean
  Scope : Scope
  Scope1 : Scope  NumInputPorts=3
  Terminator{1,3,6..7} (4 alike) : Terminator
  beforeovertaking : MATLAB Function  TreatAsAtomicUnit=on
  zoning : MATLAB Function  TreatAsAtomicUnit=on
  Out1 : Outport  OutputWhenDisabled=reset  InitialOutput=0
  wires:
  beforeovertaking/3(y3) -> Scope1/3, Logical Operator/3  "满足左后车安全距离"
  Logical Operator/1 -> Scope/1, Out1/1  "1则满足超车条件"
  beforeovertaking/1(y1) -> Scope1/1, Logical Operator/1  "满足前方纵向安全距离"
  [Tgt_lf] -> beforeovertaking/3(Tgt_lf)
  beforeovertaking/2(y2) -> Scope1/2, Logical Operator/2  "满足左前方纵向安全距离"
  [Tgt_lr] -> beforeovertaking/4(Tgt_lr)
  bus/1 -> Bus Selector2/1, Bus Selector/1
  Bus Selector2/1 -> zoning/1(Ego)  "<Ego>"
  Bus Selector2/2 -> zoning/2(Tgt)  "<Tgt>"
  Bus Selector2/3 -> zoning/3(y_line)  "<y_line>"
  [Tgt_f] -> beforeovertaking/2(Tgt_f)
  Bus Selector/1 -> beforeovertaking/1(Ego)  "<Ego>"
  Bus Selector/2 -> beforeovertaking/5(Threshold_para)  "<para>"
  zoning/5(Tgt_rf) -> Terminator6/1
  zoning/7(Egolane) -> Terminator1/1
  zoning/2(Tgt_b) -> Terminator3/1
  zoning/1(Tgt_f) -> [Tgt_f]
  zoning/6(Tgt_rr) -> Terminator7/1
  zoning/3(Tgt_lf) -> [Tgt_lf]
  zoning/4(Tgt_lr) -> [Tgt_lr]

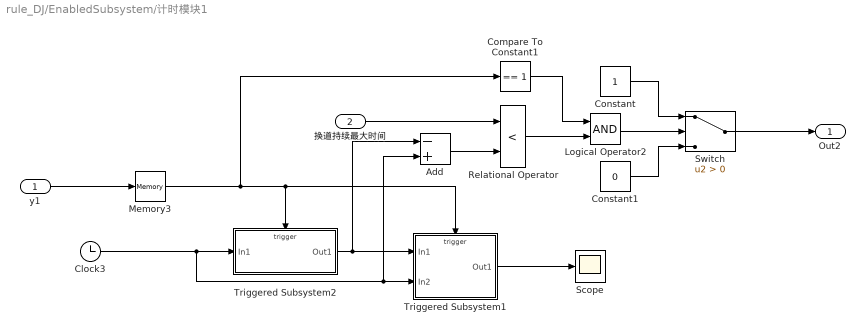
== system rule_DJ/EnabledSubsystem/计时模块1 ==
  y1 : Inport
  换道持续最大时间 : Inport  Port=2
  Add : Sum  Inputs=-+
  Clock3 : Clock
  Compare To Constant1 : simulink/Logic and Bit Operations/Compare To Constant  relop===  const=1  OutDataTypeStr=boolean
  Constant : Constant
  Constant1 : Constant  Value=0
  Logical Operator2 : Logic  AllPortsSameDT=off  OutDataTypeStr=boolean
  Memory3 : Memory
  Relational Operator : RelationalOperator  Operator=<  OutDataTypeStr=boolean  RndMeth=Simplest
  Scope : Scope
  Switch : Switch  Criteria=u2 > Threshold
  Triggered Subsystem1 : Subsystem  TreatAsAtomicUnit=on
  Triggered Subsystem2 : Subsystem  TreatAsAtomicUnit=on
  Out2 : Outport  VectorParamsAs1DForOutWhenUnconnected=off
  wires:
  Relational Operator/1 -> Logical Operator2/2
  Compare To Constant1/1 -> Logical Operator2/1
  Triggered Subsystem1/1(Out1) -> Scope/1
  Logical Operator2/1 -> Switch/2
  y1/1 -> Memory3/1
  Memory3/1 -> Compare To Constant1/1, Triggered Subsystem1/Trigger, Triggered Subsystem2/Trigger
  Add/1 -> Relational Operator/2
  Clock3/1 -> Add/2, Triggered Subsystem1/2(In2), Triggered Subsystem2/1(In1)
  Triggered Subsystem2/1(Out1) -> Add/1, Triggered Subsystem1/1(In1)
  换道持续最大时间/1 -> Relational Operator/1
  Constant/1 -> Switch/1
  Constant1/1 -> Switch/3
  Switch/1 -> Out2/1

== system rule_DJ/Subsystem2/Triggered Subsystem2 ==
  lane_Ego : Inport
  Trigger : TriggerPort  VariantControl=Variant
  Out1 : Outport  VectorParamsAs1DForOutWhenUnconnected=off
  wires:
  lane_Ego/1 -> Out1/1

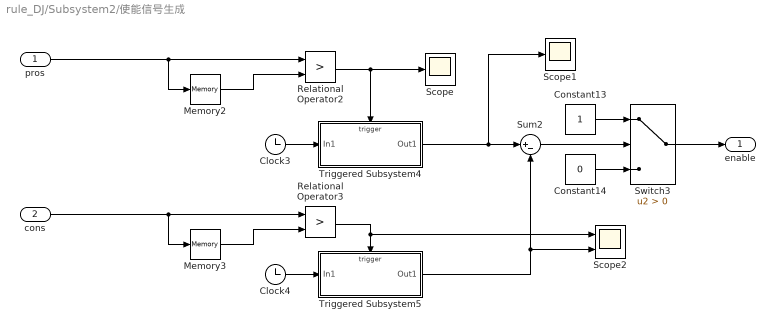
== system rule_DJ/Subsystem2/使能信号生成 ==
  pros : Inport
  cons : Inport  Port=2
  Clock3 : Clock
  Clock4 : Clock
  Constant13 : Constant
  Constant14 : Constant  Value=0
  Memory2 : Memory
  Memory3 : Memory
  Relational Operator2 : RelationalOperator  Operator=>  OutDataTypeStr=boolean  RndMeth=Simplest
  Relational Operator3 : RelationalOperator  Operator=>  OutDataTypeStr=boolean  RndMeth=Simplest
  Scope : Scope
  Scope1 : Scope
  Scope2 : Scope  NumInputPorts=2
  Sum2 : Sum  Inputs=|+-
  Switch3 : Switch  Criteria=u2 > Threshold
  Triggered Subsystem4 : Subsystem  TreatAsAtomicUnit=on
  Triggered Subsystem5 : Subsystem  TreatAsAtomicUnit=on
  enable : Outport
  wires:
  Relational Operator3/1 -> Triggered Subsystem5/Trigger, Scope2/1
  Constant14/1 -> Switch3/3
  Triggered Subsystem4/1(Out1) -> Scope1/1, Sum2/1
  Sum2/1 -> Switch3/2
  pros/1 -> Memory2/1, Relational Operator2/1
  Clock4/1 -> Triggered Subsystem5/1(In1)
  Memory3/1 -> Relational Operator3/2
  Relational Operator2/1 -> Scope/1, Triggered Subsystem4/Trigger
  Memory2/1 -> Relational Operator2/2
  Clock3/1 -> Triggered Subsystem4/1(In1)
  Triggered Subsystem5/1(Out1) -> Scope2/2, Sum2/2
  Constant13/1 -> Switch3/1
  Switch3/1 -> enable/1
  cons/1 -> Memory3/1, Relational Operator3/1

== system rule_DJ/dataset initial lane/Triggered Subsystem ==
  In1 : Inport
  Trigger : TriggerPort  VariantControl=(inherit)
  Out1 : Outport  InitialOutput=0
  wires:
  In1/1 -> Out1/1

== system rule_DJ/rule78/限速标志管理区域 ==
  note: 当车辆感知范围内没有限速标志和解除限速标志时，确定车辆是处于限速标志管理路段还是无限速标志管理路段
  Enter : Inport
  clear : Inport  Port=2
  Add : Sum  Inputs=+-
  Clock1 : Clock
  Logical Operator3 : Logic  Operator=NOT  AllPortsSameDT=off  OutDataTypeStr=boolean
  Memory : Memory
  Switch2 : Switch  Criteria=u2 > Threshold
  Triggered Subsystem : Subsystem  TreatAsAtomicUnit=on
  Triggered Subsystem3 : Subsystem  TreatAsAtomicUnit=on
  Triggered Subsystem4 : Subsystem  TreatAsAtomicUnit=on
  Triggered Subsystem5 : Subsystem  TreatAsAtomicUnit=on
  spdsign_section : Outport
  wires:
  Triggered Subsystem/1(Out1) -> Switch2/3, Triggered Subsystem3/1(In1)
  clear/1 -> Memory/1
  Triggered Subsystem5/1(Out1) -> Add/2
  Clock1/1 -> Triggered Subsystem5/1(In1), Triggered Subsystem4/1(In1)
  Switch2/1 -> spdsign_section/1
  Triggered Subsystem3/1(Out1) -> Logical Operator3/1
  Enter/1 -> Triggered Subsystem4/Trigger, Triggered Subsystem3/Enable
  Logical Operator3/1 -> Switch2/1
  Add/1 -> Switch2/2
  Triggered Subsystem4/1(Out1) -> Add/1
  Memory/1 -> Triggered Subsystem/Enable, Triggered Subsystem/1(In1), Triggered Subsystem5/Trigger

== system rule_DJ/EnabledSubsystem/EnabledSubsystem/distance ==
  bus : Inport
  Enable : EnablePort  StatesWhenEnabling=reset
  Bus Selector : BusSelector  OutputSignals=Ego,para
  Bus Selector2 : BusSelector  OutputSignals=Ego,Tgt,y_line
  Logical Operator : Logic  Operator=OR  Inputs=3  AllPortsSameDT=off  OutDataTypeStr=boolean
  Scope : Scope
  Terminator{1..4} (4 alike) : Terminator
  beforerchangelane : MATLAB Function  TreatAsAtomicUnit=on
  zoning : MATLAB Function  TreatAsAtomicUnit=on
  Out1 : Outport  OutputWhenDisabled=reset  InitialOutput=0
  wires:
  beforerchangelane/3(y3) -> Logical Operator/3  "满足右后车安全距离"
  Logical Operator/1 -> Scope/1, Out1/1  "1则满足超车条件"
  beforerchangelane/1(y1) -> Logical Operator/1  "满足前方纵向安全距离"
  beforerchangelane/2(y2) -> Logical Operator/2  "满足右前方纵向安全距离"
  zoning/6(Tgt_rr) -> beforerchangelane/3(Tgt_rr)
  zoning/3(Tgt_lf) -> Terminator3/1
  zoning/4(Tgt_lr) -> Terminator4/1
  bus/1 -> Bus Selector2/1, Bus Selector/1
  Bus Selector2/1 -> zoning/1(Ego)  "<Ego>"
  zoning/1(Tgt_f) -> beforerchangelane/1(Tgt_f)
  Bus Selector2/2 -> zoning/2(Tgt)  "<Tgt>"
  Bus Selector2/3 -> zoning/3(y_line)  "<y_line>"
  zoning/5(Tgt_rf) -> beforerchangelane/2(Tgt_rf)
  Bus Selector/1 -> beforerchangelane/4(Ego)  "<Ego>"
  Bus Selector/2 -> beforerchangelane/5(Threshold_para)  "<para>"
  zoning/2(Tgt_b) -> Terminator2/1
  zoning/7(Egolane) -> Terminator1/1

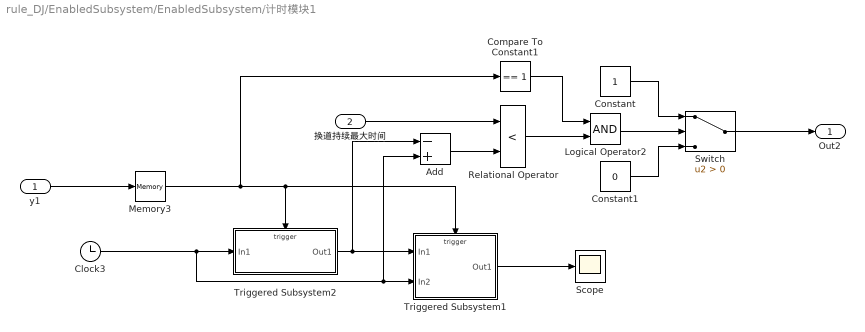
== system rule_DJ/EnabledSubsystem/EnabledSubsystem/计时模块1 ==
  y1 : Inport
  换道持续最大时间 : Inport  Port=2
  Add : Sum  Inputs=-+
  Clock3 : Clock
  Compare To Constant1 : simulink/Logic and Bit Operations/Compare To Constant  relop===  const=1  OutDataTypeStr=boolean
  Constant : Constant
  Constant1 : Constant  Value=0
  Logical Operator2 : Logic  AllPortsSameDT=off  OutDataTypeStr=boolean
  Memory3 : Memory
  Relational Operator : RelationalOperator  Operator=<  OutDataTypeStr=boolean  RndMeth=Simplest
  Scope : Scope
  Switch : Switch  Criteria=u2 > Threshold
  Triggered Subsystem1 : Subsystem  TreatAsAtomicUnit=on
  Triggered Subsystem2 : Subsystem  TreatAsAtomicUnit=on
  Out2 : Outport  VectorParamsAs1DForOutWhenUnconnected=off
  wires:
  Relational Operator/1 -> Logical Operator2/2
  Compare To Constant1/1 -> Logical Operator2/1
  Triggered Subsystem1/1(Out1) -> Scope/1
  Logical Operator2/1 -> Switch/2
  y1/1 -> Memory3/1
  Memory3/1 -> Compare To Constant1/1, Triggered Subsystem1/Trigger, Triggered Subsystem2/Trigger
  Add/1 -> Relational Operator/2
  Clock3/1 -> Add/2, Triggered Subsystem1/2(In2), Triggered Subsystem2/1(In1)
  Triggered Subsystem2/1(Out1) -> Add/1, Triggered Subsystem1/1(In1)
  换道持续最大时间/1 -> Relational Operator/1
  Constant/1 -> Switch/1
  Constant1/1 -> Switch/3
  Switch/1 -> Out2/1

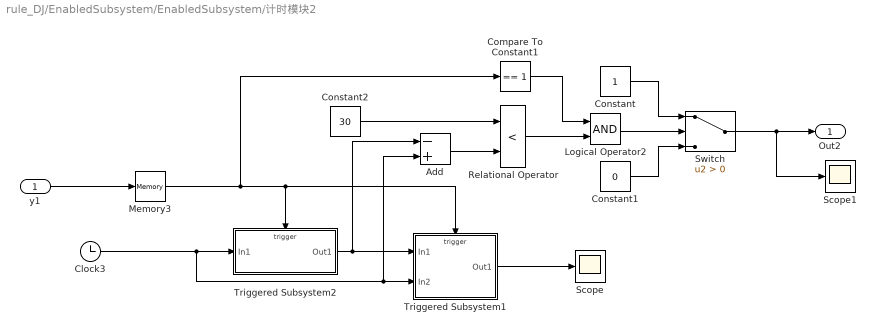
== system rule_DJ/EnabledSubsystem/EnabledSubsystem/计时模块2 ==
  y1 : Inport
  Add : Sum  Inputs=-+
  Clock3 : Clock
  Compare To Constant1 : simulink/Logic and Bit Operations/Compare To Constant  relop===  const=1  OutDataTypeStr=boolean
  Constant : Constant
  Constant1 : Constant  Value=0
  Constant2 : Constant  Value=30
  Logical Operator2 : Logic  AllPortsSameDT=off  OutDataTypeStr=boolean
  Memory3 : Memory
  Relational Operator : RelationalOperator  Operator=<  OutDataTypeStr=boolean  RndMeth=Simplest
  Scope : Scope
  Scope1 : Scope
  Switch : Switch  Criteria=u2 > Threshold
  Triggered Subsystem1 : Subsystem  TreatAsAtomicUnit=on
  Triggered Subsystem2 : Subsystem  TreatAsAtomicUnit=on
  Out2 : Outport  VectorParamsAs1DForOutWhenUnconnected=off
  wires:
  Switch/1 -> Scope1/1, Out2/1
  Constant1/1 -> Switch/3
  Constant/1 -> Switch/1
  Constant2/1 -> Relational Operator/1
  Triggered Subsystem2/1(Out1) -> Triggered Subsystem1/1(In1), Add/1
  Clock3/1 -> Triggered Subsystem2/1(In1), Triggered Subsystem1/2(In2), Add/2
  Add/1 -> Relational Operator/2
  Memory3/1 -> Triggered Subsystem2/Trigger, Triggered Subsystem1/Trigger, Compare To Constant1/1
  y1/1 -> Memory3/1
  Logical Operator2/1 -> Switch/2
  Triggered Subsystem1/1(Out1) -> Scope/1
  Compare To Constant1/1 -> Logical Operator2/1
  Relational Operator/1 -> Logical Operator2/2

== system rule_DJ/EnabledSubsystem/EnabledSubsystem1/distance ==
  bus : Inport
  Enable : EnablePort  StatesWhenEnabling=reset
  Bus Selector : BusSelector  OutputSignals=Ego,para
  Bus Selector2 : BusSelector  OutputSignals=Ego,Tgt,y_line
  Scope : Scope
  Terminator{1..6} (6 alike) : Terminator
  beforerchangelane : MATLAB Function  TreatAsAtomicUnit=on
  zoning : MATLAB Function  TreatAsAtomicUnit=on
  Out1 : Outport
  wires:
  zoning/7(Egolane) -> Terminator1/1
  zoning/2(Tgt_b) -> Terminator2/1
  Bus Selector/2 -> beforerchangelane/3(Threshold_para)  "<para>"
  Bus Selector/1 -> beforerchangelane/2(Ego)  "<Ego>"
  Bus Selector2/3 -> zoning/3(y_line)  "<y_line>"
  Bus Selector2/2 -> zoning/2(Tgt)  "<Tgt>"
  Bus Selector2/1 -> zoning/1(Ego)  "<Ego>"
  bus/1 -> Bus Selector/1, Bus Selector2/1
  zoning/4(Tgt_lr) -> beforerchangelane/1(Tgt_lr)
  zoning/3(Tgt_lf) -> Terminator3/1
  beforerchangelane/1(y3) -> Scope/1, Out1/1  "满足右后车安全距离"
  zoning/1(Tgt_f) -> Terminator4/1
  zoning/5(Tgt_rf) -> Terminator5/1
  zoning/6(Tgt_rr) -> Terminator6/1

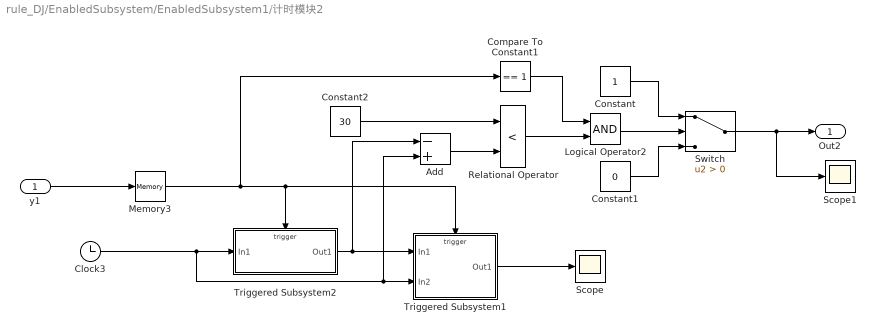
== system rule_DJ/EnabledSubsystem/EnabledSubsystem1/计时模块2 ==
  y1 : Inport
  Add : Sum  Inputs=-+
  Clock3 : Clock
  Compare To Constant1 : simulink/Logic and Bit Operations/Compare To Constant  relop===  const=1  OutDataTypeStr=boolean
  Constant : Constant
  Constant1 : Constant  Value=0
  Constant2 : Constant  Value=30
  Logical Operator2 : Logic  AllPortsSameDT=off  OutDataTypeStr=boolean
  Memory3 : Memory
  Relational Operator : RelationalOperator  Operator=<  OutDataTypeStr=boolean  RndMeth=Simplest
  Scope : Scope
  Scope1 : Scope
  Switch : Switch  Criteria=u2 > Threshold
  Triggered Subsystem1 : Subsystem  TreatAsAtomicUnit=on
  Triggered Subsystem2 : Subsystem  TreatAsAtomicUnit=on
  Out2 : Outport  VectorParamsAs1DForOutWhenUnconnected=off
  wires:
  Switch/1 -> Scope1/1, Out2/1
  Constant1/1 -> Switch/3
  Constant/1 -> Switch/1
  Constant2/1 -> Relational Operator/1
  Triggered Subsystem2/1(Out1) -> Triggered Subsystem1/1(In1), Add/1
  Clock3/1 -> Triggered Subsystem2/1(In1), Triggered Subsystem1/2(In2), Add/2
  Add/1 -> Relational Operator/2
  Memory3/1 -> Triggered Subsystem2/Trigger, Triggered Subsystem1/Trigger, Compare To Constant1/1
  y1/1 -> Memory3/1
  Logical Operator2/1 -> Switch/2
  Triggered Subsystem1/1(Out1) -> Scope/1
  Compare To Constant1/1 -> Logical Operator2/1
  Relational Operator/1 -> Logical Operator2/2

== system rule_DJ/EnabledSubsystem/Subsystem4/使能信号生成 ==
  pros : Inport
  cons : Inport  Port=2
  Clock3 : Clock
  Clock4 : Clock
  Constant13 : Constant
  Constant14 : Constant  Value=0
  Memory2 : Memory
  Memory3 : Memory
  Relational Operator2 : RelationalOperator  Operator=>  OutDataTypeStr=boolean  RndMeth=Simplest
  Relational Operator3 : RelationalOperator  Operator=>  OutDataTypeStr=boolean  RndMeth=Simplest
  Sum2 : Sum  Inputs=|+-
  Switch3 : Switch  Criteria=u2 > Threshold
  Triggered Subsystem4 : Subsystem  TreatAsAtomicUnit=on
  Triggered Subsystem5 : Subsystem  TreatAsAtomicUnit=on
  enable : Outport
  wires:
  Relational Operator3/1 -> Triggered Subsystem5/Trigger
  Constant14/1 -> Switch3/3
  Triggered Subsystem4/1(Out1) -> Sum2/1
  cons/1 -> Memory3/1, Relational Operator3/1
  Sum2/1 -> Switch3/2
  pros/1 -> Memory2/1, Relational Operator2/1
  Clock4/1 -> Triggered Subsystem5/1(In1)
  Memory3/1 -> Relational Operator3/2
  Relational Operator2/1 -> Triggered Subsystem4/Trigger
  Memory2/1 -> Relational Operator2/2
  Clock3/1 -> Triggered Subsystem4/1(In1)
  Triggered Subsystem5/1(Out1) -> Sum2/2
  Constant13/1 -> Switch3/1
  Switch3/1 -> enable/1

== system rule_DJ/EnabledSubsystem/Subsystem4/使能信号生成1 ==
  pros : Inport
  cons : Inport  Port=2
  Clock3 : Clock
  Clock4 : Clock
  Constant13 : Constant
  Constant14 : Constant  Value=0
  Memory2 : Memory
  Memory3 : Memory
  Relational Operator2 : RelationalOperator  Operator=>  OutDataTypeStr=boolean  RndMeth=Simplest
  Relational Operator3 : RelationalOperator  Operator=>  OutDataTypeStr=boolean  RndMeth=Simplest
  Sum2 : Sum  Inputs=|+-
  Switch3 : Switch  Criteria=u2 > Threshold
  Triggered Subsystem4 : Subsystem  TreatAsAtomicUnit=on
  Triggered Subsystem5 : Subsystem  TreatAsAtomicUnit=on
  enable : Outport
  wires:
  Relational Operator3/1 -> Triggered Subsystem5/Trigger
  Constant14/1 -> Switch3/3
  Triggered Subsystem4/1(Out1) -> Sum2/1
  cons/1 -> Memory3/1, Relational Operator3/1
  Sum2/1 -> Switch3/2
  pros/1 -> Memory2/1, Relational Operator2/1
  Clock4/1 -> Triggered Subsystem5/1(In1)
  Memory3/1 -> Relational Operator3/2
  Relational Operator2/1 -> Triggered Subsystem4/Trigger
  Memory2/1 -> Relational Operator2/2
  Clock3/1 -> Triggered Subsystem4/1(In1)
  Triggered Subsystem5/1(Out1) -> Sum2/2
  Constant13/1 -> Switch3/1
  Switch3/1 -> enable/1

== system rule_DJ/EnabledSubsystem/计时模块1/Triggered Subsystem1 ==
  In1 : Inport
  In2 : Inport  Port=2
  Trigger : TriggerPort  TriggerType=falling  VariantControl=Variant
  Add : Sum  Inputs=-+
  Out1 : Outport  VectorParamsAs1DForOutWhenUnconnected=off
  wires:
  Add/1 -> Out1/1
  In2/1 -> Add/2
  In1/1 -> Add/1

== system rule_DJ/EnabledSubsystem/计时模块1/Triggered Subsystem2 ==
  In1 : Inport
  Trigger : TriggerPort  VariantControl=Variant
  Out1 : Outport  InitialOutput=0  VectorParamsAs1DForOutWhenUnconnected=off
  wires:
  In1/1 -> Out1/1

== system rule_DJ/Subsystem2/使能信号生成/Triggered Subsystem4 ==
  In1 : Inport
  Trigger : TriggerPort  TriggerType=either  VariantControl=(inherit)
  Out1 : Outport
  wires:
  In1/1 -> Out1/1

== system rule_DJ/Subsystem2/使能信号生成/Triggered Subsystem5 ==
  In1 : Inport
  Trigger : TriggerPort  VariantControl=(inherit)
  Out1 : Outport
  wires:
  In1/1 -> Out1/1

== system rule_DJ/rule78/限速标志管理区域/Triggered Subsystem ==
  In1 : Inport
  Enable : EnablePort
  Out1 : Outport  VectorParamsAs1DForOutWhenUnconnected=off
  wires:
  In1/1 -> Out1/1

== system rule_DJ/rule78/限速标志管理区域/Triggered Subsystem3 ==
  In1 : Inport
  Enable : EnablePort
  Out1 : Outport  VectorParamsAs1DForOutWhenUnconnected=off
  wires:
  In1/1 -> Out1/1

== system rule_DJ/rule78/限速标志管理区域/Triggered Subsystem4 ==
  In1 : Inport
  Trigger : TriggerPort  VariantControl=(inherit)
  Out1 : Outport
  wires:
  In1/1 -> Out1/1

== system rule_DJ/rule78/限速标志管理区域/Triggered Subsystem5 ==
  In1 : Inport
  Trigger : TriggerPort  VariantControl=(inherit)
  Out1 : Outport
  wires:
  In1/1 -> Out1/1

== system rule_DJ/EnabledSubsystem/EnabledSubsystem/计时模块1/Triggered Subsystem1 ==
  In1 : Inport
  In2 : Inport  Port=2
  Trigger : TriggerPort  TriggerType=falling  VariantControl=Variant
  Add : Sum  Inputs=-+
  Out1 : Outport  VectorParamsAs1DForOutWhenUnconnected=off
  wires:
  Add/1 -> Out1/1
  In2/1 -> Add/2
  In1/1 -> Add/1

== system rule_DJ/EnabledSubsystem/EnabledSubsystem/计时模块1/Triggered Subsystem2 ==
  In1 : Inport
  Trigger : TriggerPort  VariantControl=Variant
  Out1 : Outport  InitialOutput=0  VectorParamsAs1DForOutWhenUnconnected=off
  wires:
  In1/1 -> Out1/1

== system rule_DJ/EnabledSubsystem/EnabledSubsystem/计时模块2/Triggered Subsystem1 ==
  In1 : Inport
  In2 : Inport  Port=2
  Trigger : TriggerPort  TriggerType=falling  VariantControl=Variant
  Add : Sum  Inputs=-+
  Out1 : Outport  VectorParamsAs1DForOutWhenUnconnected=off
  wires:
  In1/1 -> Add/1
  In2/1 -> Add/2
  Add/1 -> Out1/1

== system rule_DJ/EnabledSubsystem/EnabledSubsystem/计时模块2/Triggered Subsystem2 ==
  In1 : Inport
  Trigger : TriggerPort  VariantControl=Variant
  Out1 : Outport  InitialOutput=0  VectorParamsAs1DForOutWhenUnconnected=off
  wires:
  In1/1 -> Out1/1

== system rule_DJ/EnabledSubsystem/EnabledSubsystem1/计时模块2/Triggered Subsystem1 ==
  In1 : Inport
  In2 : Inport  Port=2
  Trigger : TriggerPort  TriggerType=falling  VariantControl=Variant
  Add : Sum  Inputs=-+
  Out1 : Outport  VectorParamsAs1DForOutWhenUnconnected=off
  wires:
  In1/1 -> Add/1
  In2/1 -> Add/2
  Add/1 -> Out1/1

== system rule_DJ/EnabledSubsystem/EnabledSubsystem1/计时模块2/Triggered Subsystem2 ==
  In1 : Inport
  Trigger : TriggerPort  VariantControl=Variant
  Out1 : Outport  InitialOutput=0  VectorParamsAs1DForOutWhenUnconnected=off
  wires:
  In1/1 -> Out1/1

== system rule_DJ/EnabledSubsystem/Subsystem4/使能信号生成/Triggered Subsystem4 ==
  In1 : Inport
  Trigger : TriggerPort  VariantControl=(inherit)
  Out1 : Outport
  wires:
  In1/1 -> Out1/1

== system rule_DJ/EnabledSubsystem/Subsystem4/使能信号生成/Triggered Subsystem5 ==
  In1 : Inport
  Trigger : TriggerPort  VariantControl=(inherit)
  Out1 : Outport
  wires:
  In1/1 -> Out1/1

== system rule_DJ/EnabledSubsystem/Subsystem4/使能信号生成1/Triggered Subsystem4 ==
  In1 : Inport
  Trigger : TriggerPort  VariantControl=(inherit)
  Out1 : Outport
  wires:
  In1/1 -> Out1/1

== system rule_DJ/EnabledSubsystem/Subsystem4/使能信号生成1/Triggered Subsystem5 ==
  In1 : Inport
  Trigger : TriggerPort  VariantControl=(inherit)
  Out1 : Outport
  wires:
  In1/1 -> Out1/1
